simulink model "Option_2"  (R2023b)
settings: Solver=VariableStepAuto  StartTime=0.0  StopTime=25  RelTol=1e-3
values from neighbouring files (symbols this model uses):
  A_current = current_values.(4)    [Part1.m]    (also in Part2.m = A(x))
  b1 = 1    [Part2.m]
  b2 = 1    [Part2.m]
  J1 = 100    [Part2.m]
  J2 = 1    [Part2.m]
settings Model: Creator=jessi  LastModifiedBy=jessi

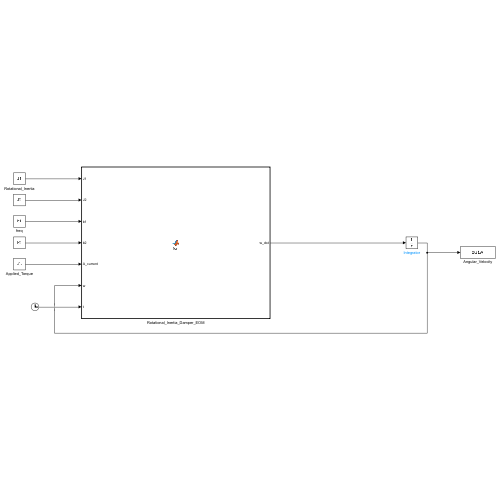
[thumbnail: Simulink's stored preview of the top-level diagram]
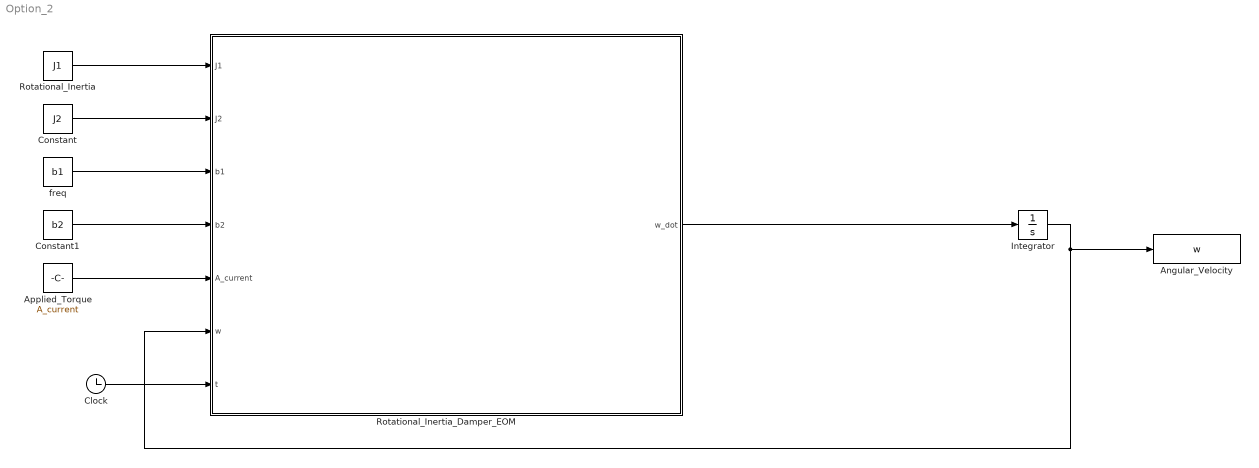
== system Option_2 ==
  Angular_Velocity : ToWorkspace  VariableName=w  SaveFormat=Timeseries  SampleTime=-1
  Applied_Torque : Constant  Value=A_current
  Clock : Clock
  Constant : Constant  Value=J2
  Constant1 : Constant  Value=b2
  Integrator : Integrator
  Rotational_Inertia : Constant  Value=J1
  Rotational_Inertia_Damper_EOM : MATLAB Function  TreatAsAtomicUnit=on
  freq : Constant  Value=b1
  wires:
  Applied_Torque/1 -> Rotational_Inertia_Damper_EOM/5(A_current)
  Clock/1 -> Rotational_Inertia_Damper_EOM/7(t)
  Rotational_Inertia_Damper_EOM/1(w_dot) -> Integrator/1
  Rotational_Inertia/1 -> Rotational_Inertia_Damper_EOM/1(J1)
  freq/1 -> Rotational_Inertia_Damper_EOM/3(b1)
  Constant/1 -> Rotational_Inertia_Damper_EOM/2(J2)
  Constant1/1 -> Rotational_Inertia_Damper_EOM/4(b2)
  Integrator/1 -> Rotational_Inertia_Damper_EOM/6(w), Angular_Velocity/1

== matlab function Option_2/Rotational_Inertia_Damper_EOM ==
  data: J1 input; w_dot output; J2 input; b1 input; b2 input; A_current input; w input; t input
function w_dot = fcn(J1,J2,b1,b2,A_current,w,t)

w_dot = (1/(J1+J2))*(A_current-(b1+b2)*w);

end
